simulink model "PEMFuelCellSystem_Cathode_cEGR_ExternalMembraneHumidifier_v01"  (R2025b)
settings: Solver=VariableStepAuto  StartTime=0.0  StopTime=100  MaxStep=0.1  RelTol=1e-3  AbsTol=1e-3
model workspace (MAT data in the model file):
  Gas_properties_block = 'PEMFuelCellSystem_Before_v01/Anode_Hydrogen_BOP/Gas Mixture
Properties'
  Gas_properties_candidates : object (value not decoded)
  T_TLU = [223.15 228.15 233.15 238.15 243.15 248.15 253.15 258.15 263.15 268.15 272.66 273.15 ... (115 elements, 1x115)]
  air_control_min_current_A = 3.8
  anode_separator_D = 0.02
  anode_separator_T0 = 20
  anode_separator_area = 0.000314159265359
  anode_separator_dp_nominal = 0.0005
  anode_separator_extra_length = 0.04
  anode_separator_laminar_fraction = 0.001
  anode_separator_length = 0.12
  anode_separator_mdot_nominal = 0.01
  anode_separator_p0 = 0.101325
  anode_separator_roughness = 1.5e-05
  anode_tube_D = 0.02
  cathode_channel_dp_nominal_MPa = 0.0368422
  cathode_channel_flow_area_m2 = 0.00403764556423
  cathode_channel_laminar_fraction = 0.5
  cathode_channel_mdot_nominal_kg_s = 0.27182
  cathode_outlet_chamber_V = 0.2
  cathode_separator_D = 0.05
  cathode_separator_T0 = 20
  cathode_separator_area = 0.00407150407905
  cathode_separator_dp_nominal = 0.002
  cathode_separator_extra_length = 0.05
  cathode_separator_laminar_fraction = 0.001
  cathode_separator_length = 0.15
  cathode_separator_mdot_nominal = 0.40798
  cathode_separator_p0 = 0.101325
  cathode_separator_roughness = 1.5e-05
  cathode_tube_D = 0.05
  cegr_comp_map_t_denom_epsilon = 1e-09
  cegr_cond_tau = 1
  cegr_inlet_mixer_p0 = 0.101325
  cegr_outlet_chamber_p0 = 0.101325
  cegr_pipe_D = 0.072
  cegr_pipe_area = 0.00407150407905
  cegr_pipe_extra_length = 0.1
  cegr_pipe_length = 0.5
  cegr_pipe_p0 = 0.101325
  cegr_pipe_roughness = 1.5e-05
  cegr_valve_max_area = 0.001
  cegr_valve_open_min_area = 1e-10
  comp_inlet_mixer_V = 0.1
  comp_mdot_corr_TLU = [0 0 0 0 0 0.28 0.26 0.24 0.22 0.2 0.56 0.52 ... (15 elements, 5x3)]
  comp_p_ratio_TLU = [1 1.5 2 2.5 3]
  comp_rpm_TLU = [0 50000 80000]
  coolant_num_layers = 20
  coolant_num_passes = 12
  coolant_tube_D = 0.05
  coolant_w_channels = 1
  drive_cycle_current = [0 0 100 100]
  drive_cycle_power = [0 0 40 40]
  drive_cycle_time = [0 0.5 60.5 600]
  drive_cycle_voltage = [427.6 427.6 410 410]
  env_RH = 0.5
  env_T = 20
  env_p = 0.101325
  env_pSat_H2O = 0.00233931818334
  env_yH20 = 0.0115436377169
  env_yO2 = 0.21
  exhaust_bp_valve_control_Ki_area_per_MPa_s = 0.002
  exhaust_bp_valve_max_area = 0.00134
  exhaust_bp_valve_open_min_area = 1e-10
  focused_anode_boundary_T_C = 20
  focused_anode_feed_p_MPa_abs = 0.3
  focused_anode_inlet_mdot_kg_s = 0.008
  focused_anode_inlet_p_MPa_abs = 0.161325
  focused_anode_outlet_p_MPa_abs = 0.101325
  focused_anode_pipe_area = 0.00246300864041
  focused_anode_pipe_extra_length = 0.1
  focused_anode_pipe_length = 1
  focused_anode_pipe_roughness = 1.5e-05
  focused_anode_yH2 = 0.9997
  focused_cathode_inlet_temperature_C = 58.9
  focused_stack_temperature_C = 80
  humidifier_bypass_mode : string (value not decoded)
  intercooler_Dh = 0.05
  intercooler_T0 = 20
  intercooler_area = 0.00785398163397
  intercooler_cond_tau = 1
  intercooler_dp_nominal = 0.005
  intercooler_extra_length = 0.05
  intercooler_laminar_fraction = 0.001
  intercooler_length = 0.25
  intercooler_mdot_nominal = 0.40798
  intercooler_p0 = 0.101325
  intercooler_roughness = 1.5e-05
  membrane_humidifier_dry_area_m2 = 0.01
  membrane_humidifier_dry_extra_length_m = 0.1
  membrane_humidifier_dry_hydraulic_diameter_m = 0.05
  membrane_humidifier_dry_length_m = 1
  membrane_humidifier_dry_roughness_m = 1.5e-05
  membrane_humidifier_heat_conductivity_W_per_m_K = 5
  membrane_humidifier_temperature_transfer_time_constant_s = 0.2
  membrane_humidifier_water_transfer_conductance_kg_s_Pa = 1e-08
  membrane_humidifier_water_transfer_time_constant_s = 0.5
  membrane_humidifier_wet_area_m2 = 0.01
  membrane_humidifier_wet_extra_length_m = 0.1
  membrane_humidifier_wet_hydraulic_diameter_m = 0.05
  membrane_humidifier_wet_length_m = 1
  membrane_humidifier_wet_roughness_m = 1.5e-05
  pSat_H2O_TLU = [0.0039376926592 0.00720321689378 0.0128411282011 0.0223441068076 0.0380050105363 0.0632733889962 0.103238678713 0.165273175188 0.259872929049 0.401739659013 0.586936061043 0.611151401419 ... (115 elements, 1x115)]
  pSat_TLU = [3379.45709837 5023.40410987 1277.63968517 0.0039376926592 3379.45809837 5023.40510987 1277.64068517 0.00720321689378 3379.45909837 5023.40610987 1277.64168517 0.0128411282011 ... (460 elements, 4x115)]
  radiator_H = 0.5
  radiator_L = 1
  radiator_N_fins = 12000
  radiator_N_tubes = 25
  radiator_W = 0.025
  radiator_air_area_fins = 11.5625
  radiator_air_area_primary = 1.223125
  radiator_cp = 910
  radiator_eta_fin = 0.7
  radiator_fin_spacing = 0.002
  radiator_gap_H = 0.0192708333333
  radiator_rho = 2700
  radiator_t_wall = 0.0001
  radiator_tube_H = 0.0015
  radiator_tube_Leq = 2.5
  routeA_air_control_mode_id = 2
  routeA_air_pid_Ki = 0.5
  routeA_air_pid_Kp = 5
  routeA_anode_inlet_pressure_MPa_abs = 0.161325
  routeA_anode_purge_enable = 1
  routeA_anode_purge_off_n2_mole_fraction = 0.1
  routeA_anode_purge_on_n2_mole_fraction = 0.5
  routeA_anode_recirculation_base_command = 0.2
  routeA_anode_recirculation_current_gain_A_inv = 0.00204081632653
  routeA_anode_rh_setpoint = 1
  routeA_backpressure_control_mode_id = 1
  routeA_cathode_humidifier_gain = 1
  routeA_cathode_rh_setpoint = 1
  routeA_cegr_enabled = 1
  routeA_cegr_valve_mode_id = 1
  routeA_command_profile = [0 0.5 60.5 600 0.101325 0.101325 0.101325 0.101325 20 20 20 20 ... (92 elements, 4x23)]
  routeA_command_profile_baseline = [0.101325 20 0.21 0.0115436377169 0.045 3 0.5 0.1613 1 1 0 70 ... (22 elements, 1x22)]
  routeA_command_profile_fields : string (value not decoded)
  routeA_command_profile_schema : string (value not decoded)
  routeA_current_default_ref_A = 28
  routeA_egr_control_Ki_area = 3.92699081699e-05
  routeA_egr_control_Kp_area = 0.000196349540849
  routeA_egr_control_mode_id = 1
  routeA_egr_target_input_mode_id = 1
  routeA_egr_valve_actuator_tau = 0.5
  routeA_egr_valve_area_direct = 3.92699081699e-06
  routeA_external_case_enabled = 0
  routeA_parameter_layer : string (value not decoded)
  routeA_stack_temperature_set_C = 80
  routeA_target_egr_ratio_comp_in = 0.02
  routeA_voltage_current_max_A = 392
  routeA_voltage_current_min_A = 0
  routeA_voltage_default_ref_V = 394.9
  routeA_voltage_pi_Ki = 0.05
  routeA_voltage_pi_Kp = 1
  separator_condensation_enabled = 1
  separator_l2_efficiency = 0.5
  separator_l2_source : string (value not decoded)
  stack_alpha = 1
  stack_area = 380
  stack_iL = 2.5
  stack_io = 2e-14
  stack_mea_cp = 870
  stack_mea_rho = 1800
  stack_num_cells = 606
  stack_num_channels = 8
  stack_t_gdl = 250
  stack_t_membrane = 125
  stack_w_channels = 1.16496474502
  tank_T = 20
  tank_V = 120
  tank_p = 70
  tank_yH2 = 0.9997
libraries: nesl_utility x57, FuelCell_lib x39, fl_lib x24, slpidlib x4
(part 6 of 6)

== system PEMFuelCellSystem_Cathode_cEGR_ExternalMembraneHumidifier_v01/Control_and_Result_Observability/Electrical_Load_Boundary/Inputs/Voltage Demand ==
  Current Command : nesl_utility/Simulink-PS Converter  PhysicalDomain=network_engine_domain  SubClassName=ps_input  LeftPortType=input  RightPortType=output  PseudoPeriodic=off  Frequencies=[]  NoiseDistribution=none  NoiseParameters=[]  Unit=A  AffineConversion=off  FilteringAndDerivatives=provide  SimscapeFilterOrder=1  InputFilterTimeConstant=0.001  UdotUserProvided=0
  Current Command Dynamics : TransferFcn  Denominator=[0.1 1]
  Raw PI Diagnostic : slpidlib/PID Controller  Controller=PI  Form=Parallel  TimeDomain=Continuous-time  UseExternalTs=off  SampleTime=-1  IntegratorMethod=Forward Euler  FilterMethod=Forward Euler  ControllerParametersSource=internal  P=routeA_voltage_pi_Kp  I=routeA_voltage_pi_Ki  UseKiTs=off  D=0  UseExternalDerivativeSource=off  N=100  UseFilter=on  TunerSelectOption=Transfer Function Based (PID Tuner App)  InitialConditionSource=internal  InitialConditionForIntegrator=0  InitialConditionForFilter=0  DifferentiatorICPrevScaledInput=0  ExternalReset=none  TrackingMode=off  Kt=1  LimitOutput=off  SatLimitsSource=internal  UpperSaturationLimit=inf  LowerSaturationLimit=-inf  LinearizeAsGain=on  AntiWindupMode=none  Kb=1  LimitIntegrator=off  UpperIntegratorSaturationLimit=inf  LowerIntegratorSaturationLimit=-inf  POutMin=[]  POutMax=[]  IOutMin=[]  IOutMax=[]  DOutMin=[]  DOutMax=[]  NOutMin=[]  NOutMax=[]  SumOutMin=[]  SumOutMax=[]  SaturationOutMin=[]  SaturationOutMax=[]  PParamMin=[]  PParamMax=[]  IParamMin=[]  IParamMax=[]  DParamMin=[]  DParamMax=[]  NParamMin=[]  NParamMax=[]  KbParamMin=[]  KbParamMax=[]  KtParamMin=[]  KtParamMax=[]  KbOutMin=[]  KbOutMax=[]  KtOutMin=[]  KtOutMax=[]  IntegratorOutMin=[]  IntegratorOutMax=[]  FilterOutMin=[]  FilterOutMax=[]  SumI1OutMin=[]  SumI1OutMax=[]  SumI2OutMin=[]  SumI2OutMax=[]  SumI3OutMin=[]  SumI3OutMax=[]  SumI4OutMin=[]  SumI4OutMax=[]  SumDOutMin=[]  SumDOutMax=[]  DifferentiatorOutMin=[]  DifferentiatorOutMax=[]  FilterDiffOutCoefMin=[]  FilterDiffOutCoefMax=[]  ReciprocalOutMin=[]  ReciprocalOutMax=[]  SumDenOutMin=[]  SumDenOutMax=[]  SumNumOutMin=[]  SumNumOutMax=[]  DivideOutMin=[]  DivideOutMax=[]  UdiffTsProdOutMin=[]  UdiffTsProdOutMax=[]  NTsProdOutMin=[]  NTsProdOutMax=[]  UintegralTsProdOutMin=[]  UintegralTsProdOutMax=[]  UngainTsProdOutMin=[]  UngainTsProdOutMax=[]  ClampingZeroOutDataTypeStr=Inherit: Inherit via back propagation  ClampingZeroOutMin=[]  ClampingZeroOutMax=[]  FilterDenConstantOutDataTypeStr=Inherit: Inherit via back propagation  FilterDenConstantOutMin=[]  FilterDenConstantOutMax=[]  PCopyOutDataTypeStr=Inherit: Inherit via back propagation  PCopyOutMin=[]  PCopyOutMax=[]  NCopyOutDataTypeStr=Inherit: Inherit via back propagation  NCopyOutMin=[]  NCopyOutMax=[]  IntegratorContinuousStateAttributes=''  IntegratorStateMustResolveToSignalObject=off  IntegratorRTWStateStorageClass=Auto  FilterContinuousStateAttributes=''  FilterStateMustResolveToSignalObject=off  FilterRTWStateStorageClass=Auto  ParallelPVariant=InternalParameters  IdealPVariant=Disabled  IVariant=InternalParameters  DVariant=Disabled  IntegratorVariant=Continuous  SatVariant=Disabled  AWVariant=Passthrough  PCopyVariant=Disabled  TRVariant=Disabled  FdbkBlocksVariant=Forward  IdealPFdbkVariant=Disabled  SatFdbkVariant=Disabled  DerivativeFilterVariant=Disabled  NVariant=Disabled  NCopyVariant=Disabled_SignalSpec  FilterICVariant=Disabled  IntegratorICVariant=InternalICs  ExternalResetVariant=Disabled  TRSumVariant=Passthrough  SumFdbkVariant=Disabled  SumVariant=Sum_PI  TsampFilterVariant=InternalTs  TsampNgainVariant=Passthrough  TsampIntegralVariant=Disabled_SignalSpec  ExternalSaturationOutDataTypeStr=Inherit: Same as second input  DerivativeSourceVariant=Disabled  PreIntVariant=InternalPreInt
  Saturation Status : RelationalOperator  Operator=~=
  Saturation Status Terminator : Terminator
  Voltage Error : Sum  Inputs=+-
  Voltage Measurement : nesl_utility/PS-Simulink Converter  PhysicalDomain=network_engine_domain  SubClassName=ps_output  LeftPortType=input  RightPortType=output  PseudoPeriodic=off  Frequencies=[]  VectorFormat=inherit  Unit=V  AffineConversion=off
  Voltage PI : slpidlib/PID Controller  Controller=PI  Form=Parallel  TimeDomain=Continuous-time  UseExternalTs=off  SampleTime=-1  IntegratorMethod=Forward Euler  FilterMethod=Forward Euler  ControllerParametersSource=internal  P=routeA_voltage_pi_Kp  I=routeA_voltage_pi_Ki  UseKiTs=off  D=0  UseExternalDerivativeSource=off  N=100  UseFilter=on  TunerSelectOption=Transfer Function Based (PID Tuner App)  InitialConditionSource=internal  InitialConditionForIntegrator=0  InitialConditionForFilter=0  DifferentiatorICPrevScaledInput=0  ExternalReset=none  TrackingMode=off  Kt=1  LimitOutput=on  SatLimitsSource=internal  UpperSaturationLimit=routeA_voltage_current_max_A  LowerSaturationLimit=routeA_voltage_current_min_A  LinearizeAsGain=on  AntiWindupMode=clamping  Kb=1  LimitIntegrator=off  UpperIntegratorSaturationLimit=inf  LowerIntegratorSaturationLimit=-inf  POutMin=[]  POutMax=[]  IOutMin=[]  IOutMax=[]  DOutMin=[]  DOutMax=[]  NOutMin=[]  NOutMax=[]  SumOutMin=[]  SumOutMax=[]  SaturationOutMin=[]  SaturationOutMax=[]  PParamMin=[]  PParamMax=[]  IParamMin=[]  IParamMax=[]  DParamMin=[]  DParamMax=[]  NParamMin=[]  NParamMax=[]  KbParamMin=[]  KbParamMax=[]  KtParamMin=[]  KtParamMax=[]  KbOutMin=[]  KbOutMax=[]  KtOutMin=[]  KtOutMax=[]  IntegratorOutMin=[]  IntegratorOutMax=[]  FilterOutMin=[]  FilterOutMax=[]  SumI1OutMin=[]  SumI1OutMax=[]  SumI2OutMin=[]  SumI2OutMax=[]  SumI3OutMin=[]  SumI3OutMax=[]  SumI4OutMin=[]  SumI4OutMax=[]  SumDOutMin=[]  SumDOutMax=[]  DifferentiatorOutMin=[]  DifferentiatorOutMax=[]  FilterDiffOutCoefMin=[]  FilterDiffOutCoefMax=[]  ReciprocalOutMin=[]  ReciprocalOutMax=[]  SumDenOutMin=[]  SumDenOutMax=[]  SumNumOutMin=[]  SumNumOutMax=[]  DivideOutMin=[]  DivideOutMax=[]  UdiffTsProdOutMin=[]  UdiffTsProdOutMax=[]  NTsProdOutMin=[]  NTsProdOutMax=[]  UintegralTsProdOutMin=[]  UintegralTsProdOutMax=[]  UngainTsProdOutMin=[]  UngainTsProdOutMax=[]  ClampingZeroOutDataTypeStr=Inherit: Inherit via back propagation  ClampingZeroOutMin=[]  ClampingZeroOutMax=[]  FilterDenConstantOutDataTypeStr=Inherit: Inherit via back propagation  FilterDenConstantOutMin=[]  FilterDenConstantOutMax=[]  PCopyOutDataTypeStr=Inherit: Inherit via back propagation  PCopyOutMin=[]  PCopyOutMax=[]  NCopyOutDataTypeStr=Inherit: Inherit via back propagation  NCopyOutMin=[]  NCopyOutMax=[]  IntegratorContinuousStateAttributes=''  IntegratorStateMustResolveToSignalObject=off  IntegratorRTWStateStorageClass=Auto  FilterContinuousStateAttributes=''  FilterStateMustResolveToSignalObject=off  FilterRTWStateStorageClass=Auto  ParallelPVariant=InternalParameters  IdealPVariant=Disabled  IVariant=InternalParameters  DVariant=Disabled  IntegratorVariant=Continuous  SatVariant=Enabled  AWVariant=ContClampingParallel  PCopyVariant=Disabled  TRVariant=Disabled  FdbkBlocksVariant=Forward  IdealPFdbkVariant=Disabled  SatFdbkVariant=Disabled  DerivativeFilterVariant=Disabled  NVariant=Disabled  NCopyVariant=Disabled_SignalSpec  FilterICVariant=Disabled  IntegratorICVariant=InternalICs  ExternalResetVariant=Disabled  TRSumVariant=Passthrough  SumFdbkVariant=Disabled  SumVariant=Sum_PI  TsampFilterVariant=InternalTs  TsampNgainVariant=Passthrough  TsampIntegralVariant=Disabled_SignalSpec  ExternalSaturationOutDataTypeStr=Inherit: Same as second input  DerivativeSourceVariant=Disabled  PreIntVariant=InternalPreInt
  Voltage Reference : FromWorkspace  VariableName=[drive_cycle_time, drive_cycle_voltage]
  i : PMIOPort  Side=Left
  v : PMIOPort  Port=2  Side=Left
  tag scope: i_stack=global, v_stack=global
  wires:
  Current Command Dynamics/1 -> [i_stack], Current Command/1  "routeA_voltage_current_cmd_A"
  Voltage PI/1 -> Current Command Dynamics/1, Saturation Status/2  "routeA_voltage_current_cmd_limited_A"
  Voltage Error/1 -> Raw PI Diagnostic/1, Voltage PI/1  "routeA_voltage_control_error_V"
  Voltage Reference/1 -> Voltage Error/2  "routeA_voltage_ref_V"
  Voltage Measurement/1 -> Voltage Error/1, [v_stack]
  Raw PI Diagnostic/1 -> Saturation Status/1  "routeA_voltage_current_cmd_raw_A"
  Saturation Status/1 -> Saturation Status Terminator/1  "routeA_voltage_current_saturated"
  connections:
  v/RConn1 -- Voltage Measurement/LConn1
  Current Command/RConn1 -- i/RConn1

== matlab function PEMFuelCellSystem_Cathode_cEGR_ExternalMembraneHumidifier_v01/Cathode_Exhaust_and_Backpressure/CathodeOutlet_Observability/SeparatorOrCondensation ==
  data: p_MPa input; m_water_sep output; T_degC input; y_i input; egr_mdot input; exhaust_mdot input
function m_water_sep = SeparatorOrCondensation(p_MPa,T_degC,y_i,egr_mdot,exhaust_mdot)
%#codegen
% L2 saturation-excess estimator. Source: l2_saturation_excess_estimator.
p = max(double(p_MPa), 1e-6);
T = double(T_degC);
if T > 200
    Tc = T - 273.15;
else
    Tc = T;
end
Tc = min(max(Tc, -40), 120);
if numel(y_i) >= 4
    yH2O = max(double(y_i(4)), 0);
else
    yH2O = 0;
end
pSat_kPa = 0.61121 * exp((18.678 - Tc/234.5) * (Tc/(257.14 + Tc)));
pSat_MPa = max(pSat_kPa * 1e-3, 1e-9);
ySat = min(max(pSat_MPa / p, 0), 1);
excess = max(yH2O - ySat, 0);
mdotTotal = max(double(egr_mdot), 0) + max(double(exhaust_mdot), 0);
m_water_sep = mdotTotal * excess;
end
